simulink subsystem "VehicleElectroThermal"  (R2023a)
settings: Solver=VariableStepAuto  StartTime=0.0  StopTime=10.0  RelTol=1e-3
undefined symbols (not defined in the file): battery, cabin_T_init, coolant_pipe_D, coolant_valve_D_ratio_max, coolant_valve_D_ratio_min, coolant_valve_displacement, vehicleThermal
libraries: fl_lib x199, nesl_utility x54, SimscapeFluids_lib x15, ee_lib x9, sdl_lib x8, slpidlib x3, simulink x2, EmotorLib x2, BatteryCurrentManagement x1
(part 2 of 6)

== system VehicleElectroThermal/DCDC ==
  Coolant Jacket : SimscapeFluids_lib/Thermal Liquid/Pipes & Fittings/Pipe (TL)  dynamic_compressibility=1  inertia=0  num_segments=1  pipe_length=0.2 m  cross_section_geometry=fluids.thermal_liquid.pipes_fittings.enum.CrossSectionGeometry.Custom  pipe_diameter=0.1 m  pipe_inner_diameter=0.05 m  pipe_outer_diameter=0.1 m  pipe_width=0.1 m  pipe_height=0.1 m  pipe_major_axis=0.1 m  pipe_minor_axis=0.05 m  pipe_side=0.1 m  pipe_angle=30 deg  area=pi * vehicleThermal.coolant_channel_D^2 / 4 m^2  Dh=vehicleThermal.coolant_channel_D m  wall_spec=1  wall_compliance=1.2e-6 m/MPa  wall_time_constant=0.01 s  elevation_spec=foundation.enum.constant_variable.constant  elevation_gain=0 m  g=9.81 m/s^2  pressure_loss_spec=1  local_pressure_loss_spec=fluids.thermal_liquid.pipes_fittings.enum.LocalLossSpec.AggregateLength  length_add=0 m  loss_coefficient=0.1  roughness_spec=fluids.thermal_liquid.pipes_fittings.enum.RoughnessSpec.Custom  roughness=1.5e-5 m  Re_friction_TLU=[ 400 1000 1.5e+3 3e+3 4e+3 6e+3 1e+4 2e+4 4e+4 6e+4 1e+5 1e+8 ]  friction_factor_TLU=[ 0.264 0.112 0.07099999999999999 0.0417 0.0387 0.0268 0.025 0.0232 0.0226 0.022 0.0214 0.0214 ]  shape_factor=64  Re_lam=100  Re_tur=500  mdot_nominal=[ 0.1 1 ] kg/s  p_diff_nominal=[ 0.001 0.01 ] MPa  mdot_threshold=1e-6 kg/s  heat_transfer_spec=4  mdot_nominal_heat=[ 0.1 1 ] kg/s  T_in_nominal=[ 293.15 293.15 ] K  T_out_nominal=[ 300 300 ] K  p_in_nominal_heat=[ 0.101325 0.101325 ] MPa  T_wall_nominal=[ 303.15 303.15 ] K  a_coeff=0.3  b_Re_power=0.8  c_Pr_power=0.33  Nu_lam=3.66  Re_Colburn_TLU=[ 100 150 1000 ]  Colburn_factor_TLU=[ 0.019 0.013 0.002 ]  Re_Nu_TLU=[ 100 150 1000 ]  Pr_Nu_TLU=[ 1 10 ]  Nu_TLU=[ 3.72 4.21; 3.75 4.44; 4.21 7.15 ]  p0_vec=vehicleThermal.coolant_p_init MPa  T0_vec=vehicleThermal.coolant_T_init K  mdot0=0.1 kg/s
  DC-DC Converter mass : fl_lib/Thermal/Thermal Elements/Thermal Mass  mass_type=foundation.enum.constant_variable.constant  mass=1 kg  sp_heat=447 J/kg/K  mass_min=1e-6 kg  num_ports=foundation.enum.numPorts2.one  m_specify=off  m_priority=High  m=1 kg  m_nominal_specify=off  m_nominal_unit=kg  m_nominal_value=1  T_specify=on  T_priority=High  T=vehicleThermal.coolant_T_init K  T_nominal_specify=off  T_nominal_unit=K  T_nominal_value=1  Q_specify=off  Q_priority=None  Q=0 W  Q_nominal_specify=off  Q_nominal_unit=W  Q_nominal_value=1
  DC-DC Converter : ee_lib/Semiconductors & Converters/Converters/DC-DC Converter  Vref_option=ee.enum.converters.voltageref.internal  v_ref=100 V  P_rated=10000 W  droop_enabled=false  droop_param=ee.enum.converters.droop.value  droop=0.1 V/A  droop_percent=2  Vref_droop=10 V  reversible=ee.enum.converters.directionality.unidirectional  G_diode=1e-8 1/Ohm  P_fixed=1 W  losses_option=ee.enum.converters.lossesOption.proportionalToSquaredCurrent  eff_rated=80  tableOption=ee.enum.converters.lossTableOptionThermal.currentTemp  i_eff_vec=[-2, -1, 1, 2] A  v_eff_vec=[15, 30, 45] V  eff_vec=[66, 76, 80, 74]  eff_2D_table=[66, 66, 66; 76, 76, 76; 80, 80, 80; 74, 74, 74]  model_dynamics=ee.enum.converters.dynamics.yes  tau=0.02 s  v_ini=10 V  v1_min=1 V  R1=1000 Ohm  R2=1000 Ohm  enable_fault=simscape.enum.onoff.off  fault_condition=ee.enum.faults.faultInputCondition.greaterThan  fault_threshold=0.5  T_eff_vec=[280, 300, 320] K  eff_3D_table=repmat([66; 76; 80; 74], 1, 3, 3)  thermal_mass=100 J/K  initial_temperature=298.15 K
      settings: InternalSimscapePortConfiguration="{\"Bottom\":[],\"Left\":[{\"id\":\"p1\",\"label\":\"1+\",\"type\":\"foundation.electrical.electrical\"},{\"id\":\"n1\",\"label\":\"1-\",\"type\":\"foundation.electrical.electrical\"}],\"Right\":[{\"id\":\"p2\",\"label\":\"2+\",\"type\":\"foundation.electrical.electrical\"},{\"id\":\"n2\",\"label\":\"2-\",\"type\":\"foundation.electrical.electrical\"}],\"Top\":[]}"
  Electrical Reference : fl_lib/Electrical/Electrical Elements/Electrical Reference
  Electrical Reference1 : fl_lib/Electrical/Electrical Elements/Electrical Reference
  Flow Resistance (TL) : fl_lib/Thermal Liquid/Elements/Flow Resistance (TL)  delta_p_nominal=2e-3 MPa  mdot_nominal=0.02 kg/s  area=pi * vehicleThermal.coolant_pipe_D^2 / 4 m^2  laminar_fraction=1e-3
  Flow Resistance (TL)1 : fl_lib/Thermal Liquid/Elements/Flow Resistance (TL)  delta_p_nominal=1e-5 MPa  mdot_nominal=0.02 kg/s  area=pi * vehicleThermal.coolant_pipe_D^2 / 4 m^2  laminar_fraction=1e-3
  Heat Flow Source : fl_lib/Thermal/Thermal Sources/Controlled Heat Flow Rate Source
  PS Constant : fl_lib/Physical Signals/Sources/PS Constant  constant=0
  Thermal Reference : fl_lib/Thermal/Thermal Elements/Thermal Reference
  LV : PMIOPort  Side=Right
  B : PMIOPort  Port=2  Side=Right
  HV : PMIOPort  Port=3  Side=Right
  A : PMIOPort  Port=4  Side=Right
  connections:
  HV/RConn1 -- DC-DC Converter/LConn1
  DC-DC Converter/RConn1 -- LV/RConn1
  Coolant Jacket/LConn2 -- Heat Flow Source/LConn1 -- DC-DC Converter mass/LConn1
  Flow Resistance (TL)1/LConn1 -- A/RConn1
  DC-DC Converter/LConn2 -- Electrical Reference1/LConn1
  Flow Resistance (TL)1/RConn1 -- Coolant Jacket/RConn1
  Electrical Reference/LConn1 -- DC-DC Converter/RConn2
  Flow Resistance (TL)/LConn1 -- Coolant Jacket/LConn1
  Flow Resistance (TL)/RConn1 -- B/RConn1
  Thermal Reference/LConn1 -- Heat Flow Source/RConn2
  PS Constant/RConn1 -- Heat Flow Source/RConn1

== system VehicleElectroThermal/Driveline ==
  s : Inport
  Brake Rear : sdl_lib/Brakes & Detents/Rotational/Disc Brake  r_mean=150 mm  bore=10 mm  n_pads=2  thermal_port=simscape.enum.thermaleffects.omit  mu_static=0.9  mu_coulomb=0.7  temperature_TLU=[280, 300, 320] K  mu_static_TLU=[.9, .8, .7]  mu_coulomb_TLU=[.8, .7, .6]  brkwy_vel=0.1 rad/s  visc_coef=0 N*m*s/rad  enable_faults=simscape.enum.onoff.off  faulted_pressure=0 bar  external_fault=simscape.enum.onoff.off  temporal_fault=simscape.enum.onoff.off  fault_time=5 s  report_fault=simscape.enum.assert.action.none  thermal_mass=50 kJ/K  temperature_specify=off  temperature_priority=High  temperature=300 K  temperature_nominal_specify=off  temperature_nominal_unit=K  temperature_nominal_value=1
  PS-Simulink Converter1 : nesl_utility/PS-Simulink Converter  PhysicalDomain=network_engine_domain  SubClassName=ps_output  LeftPortType=input  RightPortType=output  PseudoPeriodic=off  Frequencies=[]  VectorFormat=inherit  Unit=km/hr  AffineConversion=off
  Simulink-PS Converter1 : nesl_utility/Simulink-PS Converter  PhysicalDomain=network_engine_domain  SubClassName=ps_input  LeftPortType=input  RightPortType=output  PseudoPeriodic=off  Frequencies=[]  NoiseDistribution=none  NoiseParameters=[]  Unit=1  AffineConversion=off  FilteringAndDerivatives=provide  SimscapeFilterOrder=1  InputFilterTimeConstant=0.001  UdotUserProvided=0
  Tire FL : sdl_lib/Tires & Vehicles/Tire (Magic Formula)  parameterization=sdl.enum.magic_tire_model.peak  F_z1=3000 N  F_x1=3500 N  kappa1=10  B_m=10  C_m=1.9  D_m=1  E_m=0.97  fz0=4000 N  p_Cx=1.685  p_Dx=[1.21, -.037]  p_Ex=[.344, .095, -.02, 0]  p_Kx=[21.51, -.163, .245]  p_Hx=[-.002, .002]  p_Vx=[0, 0]  rolling_radius_model=sdl.enum.RollingRadiusParameterization.Constant  r_e="vehicle.tireRollingRadius_cm  cm"  r_0=0.3 m  breff=8.39  dreff=0.26  freff=0.074  q_re0=0.99  q_v1=0.008  longvl=17 m/s  cz=5e5 N/m  model_resistance=simscape.enum.onoff.off  resistance_model=sdl.enum.rollingResistanceParameterization.constant  coeff=0.015  p_tire=250e3 Pa  alpha=-0.003  beta=0.97  coeff_a=84e-4  coeff_b=6.2e-4 s/m  coeff_c=1.6e-4 s^2/m^2  p_tire0=240e3 Pa  fz0_resistance=4000 N  vH0=16 m/s  q_Sy=[.0082, 0, .0014, .001, 0, 0, 1.08, -.5]  v_thr=0.001 m/s  enable_scaling_coefficients=false  lfzO=1  lcx=1  lmux=1  lex=1  lkx=1  lhx=1  lvx=1  lmy=1  model_compliance=sdl.enum.compliance.off  stiffness=1e6 N/m  damping=1000 N*s/m  model_inertia=sdl.enum.model_inertia.off  inertia=1 kg*m^2  initial_velocity=0 rad/s  vxlow=0.1 m/s  v_tr_thr=0.1*(0.1) m/s  kpumin=-1e5  kpumax=1e5
  Tire FR : sdl_lib/Tires & Vehicles/Tire (Magic Formula)  parameterization=sdl.enum.magic_tire_model.peak  F_z1=3000 N  F_x1=3500 N  kappa1=10  B_m=10  C_m=1.9  D_m=1  E_m=0.97  fz0=4000 N  p_Cx=1.685  p_Dx=[1.21, -.037]  p_Ex=[.344, .095, -.02, 0]  p_Kx=[21.51, -.163, .245]  p_Hx=[-.002, .002]  p_Vx=[0, 0]  rolling_radius_model=sdl.enum.RollingRadiusParameterization.Constant  r_e="vehicle.tireRollingRadius_cm  cm"  r_0=0.3 m  breff=8.39  dreff=0.26  freff=0.074  q_re0=0.99  q_v1=0.008  longvl=17 m/s  cz=5e5 N/m  model_resistance=simscape.enum.onoff.off  resistance_model=sdl.enum.rollingResistanceParameterization.constant  coeff=0.015  p_tire=250e3 Pa  alpha=-0.003  beta=0.97  coeff_a=84e-4  coeff_b=6.2e-4 s/m  coeff_c=1.6e-4 s^2/m^2  p_tire0=240e3 Pa  fz0_resistance=4000 N  vH0=16 m/s  q_Sy=[.0082, 0, .0014, .001, 0, 0, 1.08, -.5]  v_thr=0.001 m/s  enable_scaling_coefficients=false  lfzO=1  lcx=1  lmux=1  lex=1  lkx=1  lhx=1  lvx=1  lmy=1  model_compliance=sdl.enum.compliance.off  stiffness=1e6 N/m  damping=1000 N*s/m  model_inertia=sdl.enum.model_inertia.off  inertia=1 kg*m^2  initial_velocity=0 rad/s  vxlow=0.1 m/s  v_tr_thr=0.1*(0.1) m/s  kpumin=-1e5  kpumax=1e5
  Tire RL : sdl_lib/Tires & Vehicles/Tire (Magic Formula)  parameterization=sdl.enum.magic_tire_model.peak  F_z1=3000 N  F_x1=3500 N  kappa1=10  B_m=10  C_m=1.9  D_m=1  E_m=0.97  fz0=4000 N  p_Cx=1.685  p_Dx=[1.21, -.037]  p_Ex=[.344, .095, -.02, 0]  p_Kx=[21.51, -.163, .245]  p_Hx=[-.002, .002]  p_Vx=[0, 0]  rolling_radius_model=sdl.enum.RollingRadiusParameterization.Constant  r_e="vehicle.tireRollingRadius_cm  cm"  r_0=0.3 m  breff=8.39  dreff=0.26  freff=0.074  q_re0=0.99  q_v1=0.008  longvl=17 m/s  cz=5e5 N/m  model_resistance=simscape.enum.onoff.off  resistance_model=sdl.enum.rollingResistanceParameterization.constant  coeff=0.015  p_tire=250e3 Pa  alpha=-0.003  beta=0.97  coeff_a=84e-4  coeff_b=6.2e-4 s/m  coeff_c=1.6e-4 s^2/m^2  p_tire0=240e3 Pa  fz0_resistance=4000 N  vH0=16 m/s  q_Sy=[.0082, 0, .0014, .001, 0, 0, 1.08, -.5]  v_thr=0.001 m/s  enable_scaling_coefficients=false  lfzO=1  lcx=1  lmux=1  lex=1  lkx=1  lhx=1  lvx=1  lmy=1  model_compliance=sdl.enum.compliance.off  stiffness=1e6 N/m  damping=1000 N*s/m  model_inertia=sdl.enum.model_inertia.off  inertia=1 kg*m^2  initial_velocity=0 rad/s  vxlow=0.1 m/s  v_tr_thr=0.1*(0.1) m/s  kpumin=-1e5  kpumax=1e5
  Tire RR : sdl_lib/Tires & Vehicles/Tire (Magic Formula)  parameterization=sdl.enum.magic_tire_model.peak  F_z1=3000 N  F_x1=3500 N  kappa1=10  B_m=10  C_m=1.9  D_m=1  E_m=0.97  fz0=4000 N  p_Cx=1.685  p_Dx=[1.21, -.037]  p_Ex=[.344, .095, -.02, 0]  p_Kx=[21.51, -.163, .245]  p_Hx=[-.002, .002]  p_Vx=[0, 0]  rolling_radius_model=sdl.enum.RollingRadiusParameterization.Constant  r_e="vehicle.tireRollingRadius_cm  cm"  r_0=0.3 m  breff=8.39  dreff=0.26  freff=0.074  q_re0=0.99  q_v1=0.008  longvl=17 m/s  cz=5e5 N/m  model_resistance=simscape.enum.onoff.off  resistance_model=sdl.enum.rollingResistanceParameterization.constant  coeff=0.015  p_tire=250e3 Pa  alpha=-0.003  beta=0.97  coeff_a=84e-4  coeff_b=6.2e-4 s/m  coeff_c=1.6e-4 s^2/m^2  p_tire0=240e3 Pa  fz0_resistance=4000 N  vH0=16 m/s  q_Sy=[.0082, 0, .0014, .001, 0, 0, 1.08, -.5]  v_thr=0.001 m/s  enable_scaling_coefficients=false  lfzO=1  lcx=1  lmux=1  lex=1  lkx=1  lhx=1  lvx=1  lmy=1  model_compliance=sdl.enum.compliance.off  stiffness=1e6 N/m  damping=1000 N*s/m  model_inertia=sdl.enum.model_inertia.off  inertia=1 kg*m^2  initial_velocity=0 rad/s  vxlow=0.1 m/s  v_tr_thr=0.1*(0.1) m/s  kpumin=-1e5  kpumax=1e5
  Vehicle Body : sdl_lib/Tires & Vehicles/Vehicle Body  mass=vehicle.vehMass_kg kg  n_w=2  x_f=1.4 m  x_r=1.6 m  y_c=0.5 m  mass_var=simscape.enum.onoff.off  g=9.81 m/s^2  liftoff_warning=simscape.enum.onoff.off  area=3 m^2  Cd=0.4  rho=1.18 kg/m^3  model_pitch=simscape.enum.onoff.off  inertia=4000 kg*m^2  suspension_model=sdl.enum.linearTLU.linear  k_f=1e4 N/m  b_f=1e4 N*s/m  k_r=1e4 N/m  b_r=1e4 N*s/m  k_f_TLU=[-2000, -1000, 0, 1000, 2000] N  x_f_TLU=[-.4, -.2, 0, .2, .4] m  b_f_TLU=[-200, -100, 0, 100, 200] N  v_f_TLU=[-4, -2, 0, 2, 4] m/s  k_r_TLU=[-2000, -1000, 0, 1000, 2000] N  x_r_TLU=[-.4, -.2, 0, .2, .4] m  b_r_TLU=[-200, -100, 0, 100, 200] N  v_r_TLU=[-4, -2, 0, 2, 4] m/s  interp_method=simscape.enum.interpolation.linear  extrap_method=simscape.enum.extrapolation.linear  model_hardstop=simscape.enum.onoff.off  upper_bound_f=.25 m  lower_bound_f=-.25 m  stop_k_f=1e6 N/m  stop_b_f=150 N*s/m  upper_bound_r=.25 m  lower_bound_r=-.25 m  stop_k_r=1e6 N/m  stop_b_r=150 N*s/m  initial_pitch=0 rad  initial_pitch_rate=0 rad/s  v_specify=on  v_priority=High  v=0 kph  v_nominal_specify=on  v_nominal_unit=m/s  v_nominal_value=1
  FA : PMIOPort  Side=Left
  RA : PMIOPort  Port=2  Side=Right
  Bus Element Out : Outport  PortName=m  Element=VehSpd
  wires:
  s/1 -> [BrkCmd]
  PS-Simulink Converter1/1 -> Bus Element Out/1  "VehSpd"
  [BrkCmd] -> Simulink-PS Converter1/1
  connections:
  Tire FL/LConn1 -- Tire FR/LConn1 -- Vehicle Body/RConn2
  Tire RR/LConn1 -- Vehicle Body/RConn1 -- Tire RL/LConn1
  PS-Simulink Converter1/LConn1 -- Vehicle Body/LConn2
  Tire FR/LConn2 -- FA/RConn1 -- Tire FL/LConn2
  Brake Rear/LConn2 -- RA/RConn1 -- Tire RR/LConn2 -- Tire RL/LConn2
  Tire FL/RConn2 -- Vehicle Body/LConn1 -- Tire RR/RConn2 -- Tire RL/RConn2 -- Tire FR/RConn2
  Simulink-PS Converter1/RConn1 -- Brake Rear/LConn1

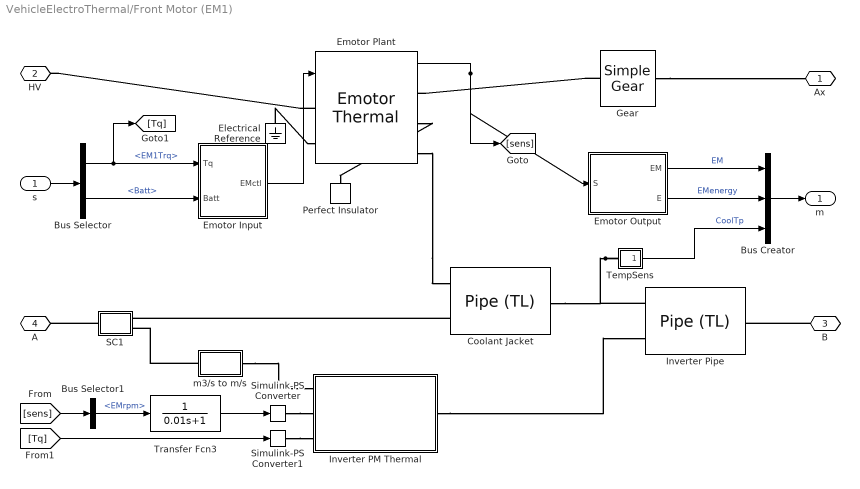
== system VehicleElectroThermal/Front Motor (EM1) ==
  s : Inport
  Bus Creator : BusCreator  Inputs=3
  Bus Selector : BusSelector  OutputSignals=EM1Trq,Batt
  Bus Selector1 : BusSelector  OutputSignals=EMrpm
  Coolant Jacket : SimscapeFluids_lib/Thermal Liquid/Pipes & Fittings/Pipe (TL)  dynamic_compressibility=1  inertia=0  num_segments=1  pipe_length=0.4 m  cross_section_geometry=fluids.thermal_liquid.pipes_fittings.enum.CrossSectionGeometry.Custom  pipe_diameter=0.1 m  pipe_inner_diameter=0.05 m  pipe_outer_diameter=0.1 m  pipe_width=0.1 m  pipe_height=0.1 m  pipe_major_axis=0.1 m  pipe_minor_axis=0.05 m  pipe_side=0.1 m  pipe_angle=30 deg  area=4 * pi * vehicleThermal.coolant_channel_D^2 / 4 m^2  Dh=vehicleThermal.coolant_channel_D m  wall_spec=1  wall_compliance=1.2e-6 m/MPa  wall_time_constant=0.01 s  elevation_spec=foundation.enum.constant_variable.constant  elevation_gain=0 m  g=9.81 m/s^2  pressure_loss_spec=1  local_pressure_loss_spec=fluids.thermal_liquid.pipes_fittings.enum.LocalLossSpec.AggregateLength  length_add=20 * vehicleThermal.coolant_channel_D * 4 m  loss_coefficient=0.1  roughness_spec=fluids.thermal_liquid.pipes_fittings.enum.RoughnessSpec.Custom  roughness=1.5e-5 m  Re_friction_TLU=[ 400 1000 1.5e+3 3e+3 4e+3 6e+3 1e+4 2e+4 4e+4 6e+4 1e+5 1e+8 ]  friction_factor_TLU=[ 0.264 0.112 0.07099999999999999 0.0417 0.0387 0.0268 0.025 0.0232 0.0226 0.022 0.0214 0.0214 ]  shape_factor=64  Re_lam=100  Re_tur=500  mdot_nominal=[ 0.1 1 ] kg/s  p_diff_nominal=[ 0.001 0.01 ] MPa  mdot_threshold=1e-6 kg/s  heat_transfer_spec=4  mdot_nominal_heat=[ 0.1 1 ] kg/s  T_in_nominal=[ 293.15 293.15 ] K  T_out_nominal=[ 300 300 ] K  p_in_nominal_heat=[ 0.101325 0.101325 ] MPa  T_wall_nominal=[ 303.15 303.15 ] K  a_coeff=0.3  b_Re_power=0.8  c_Pr_power=0.33  Nu_lam=3.66  Re_Colburn_TLU=[ 100 150 1000 ]  Colburn_factor_TLU=[ 0.019 0.013 0.002 ]  Re_Nu_TLU=[ 100 150 1000 ]  Pr_Nu_TLU=[ 1 10 ]  Nu_TLU=[ 3.72 4.21; 3.75 4.44; 4.21 7.15 ]  p0_vec=vehicleThermal.coolant_p_init MPa  T0_vec=vehicleThermal.coolant_T_init K  mdot0=0.1 kg/s
  Electrical Reference : fl_lib/Electrical/Electrical Elements/Electrical Reference
  Emotor Input : Subsystem
  Emotor Output : Subsystem
  Emotor Plant : EmotorLib/Emotor Thermal  InitTemp=vehicleThermal.coolant_T_init  IronSpHeat=electricDrive.IronSpHeat  CopperSpHeat=electricDrive.CopperSpHeat  IronThConductivity=electricDrive.IronThConductivity  GrossToothMass=electricDrive.MotorThermal.GrossToothMass  WindingMass=electricDrive.MotorThermal.WindingMass  max_torque=electricDrive.max_torque  max_power=electricDrive.max_power  Tctc=electricDrive.Tctc  spMat=electricDrive.motor_loss_map.spMat  tqMat=electricDrive.motor_loss_map.tqMat  lossMat=electricDrive.motor_loss_map.lossMat  StatorBackIronMass=electricDrive.MotorThermal.StatorBackIronMass  StatorRootDia=electricDrive.MotorThermal.StatorRootDia  stator_od=electricDrive.MotorThermal.stator_od  StatorWindingOhArea=electricDrive.MotorThermal.StatorWindingOhArea  Bridgemass=electricDrive.MotorThermal.Bridgemass  rotor_od=electricDrive.MotorThermal.rotor_od  rotorStackLength=electricDrive.MotorThermal.rotorStackLength  RotorBackIronMass=electricDrive.MotorThermal.RotorBackIronMass  RotorAreaER=electricDrive.MotorThermal.RotorAreaER  RotorAreaCyl=electricDrive.MotorThermal.RotorAreaCyl
  Gear : sdl_lib/Gears/Simple Gear  ratio=10/3  rotation_direction=sdl.enum.shaftOutputDirection.same  friction_model=sdl.enum.gear_efficiencies_load.off  T_noload=0.1 N*m  T_nom=5 N*m  efficiency_nom=0.8  efficiency=0.8  temperature_TLU=[280, 300, 320] K  load_TLU=[1, 5, 10] N*m  efficiency_TLU=[.95, .9, .85]  efficiency_TLU2=[.85, .8, .75; .95, .9, .85; .85, .8, .7]  w_thr=0.01 rad/s  pwr_thr=0.001 W  enable_backlash=false  hardstop_model=simscape.enum.hardstop.smooth  backlash_distance=1e-3 mm  r_base=0.1 m  transition=1e-4 mm  backlash_stiffness=1e7 N/m  backlash_damping=1e6 N*s/m  coeff_rest=0  v_tol=0.001 m/s  f_tol=0 N  mu_visc=[0, 0] N*m*s/rad  enable_faults=simscape.enum.onoff.off  efficiency_fault=0.05  external_fault=simscape.enum.onoff.off  temporal_fault=simscape.enum.onoff.off  fault_time=5 s  fault_angles=pi / 12 rad  report_fault=simscape.enum.assert.action.none  thermal_mass=50 J/K  temperature_specify=off  temperature_priority=High  temperature=300 K  temperature_nominal_specify=off  temperature_nominal_unit=K  temperature_nominal_value=1  x_backlash_specify=off  x_backlash_priority=None  x_backlash=0 mm  x_backlash_nominal_specify=off  x_backlash_nominal_unit=mm  x_backlash_nominal_value=1  f_hardstop_specify=off  f_hardstop_priority=None  f_hardstop=0 N  f_hardstop_nominal_specify=off  f_hardstop_nominal_unit=N  f_hardstop_nominal_value=1  v_backlash_specify=off  v_backlash_priority=None  v_backlash=0 m/s  v_backlash_nominal_specify=off  v_backlash_nominal_unit=m/s  v_backlash_nominal_value=1
  Inverter PM Thermal : Subsystem
  Inverter Pipe : SimscapeFluids_lib/Thermal Liquid/Pipes & Fittings/Pipe (TL)  dynamic_compressibility=1  inertia=0  num_segments=1  pipe_length=0.4 m  cross_section_geometry=fluids.thermal_liquid.pipes_fittings.enum.CrossSectionGeometry.Custom  pipe_diameter=0.1 m  pipe_inner_diameter=0.05 m  pipe_outer_diameter=0.1 m  pipe_width=0.1 m  pipe_height=0.1 m  pipe_major_axis=0.1 m  pipe_minor_axis=0.05 m  pipe_side=0.1 m  pipe_angle=30 deg  area=4 * pi * vehicleThermal.coolant_channel_D^2 / 4 m^2  Dh=vehicleThermal.coolant_channel_D m  wall_spec=1  wall_compliance=1.2e-6 m/MPa  wall_time_constant=0.01 s  elevation_spec=foundation.enum.constant_variable.constant  elevation_gain=0 m  g=9.81 m/s^2  pressure_loss_spec=1  local_pressure_loss_spec=fluids.thermal_liquid.pipes_fittings.enum.LocalLossSpec.AggregateLength  length_add=20 * vehicleThermal.coolant_channel_D * 4 m  loss_coefficient=0.1  roughness_spec=fluids.thermal_liquid.pipes_fittings.enum.RoughnessSpec.Custom  roughness=1.5e-5 m  Re_friction_TLU=[ 400 1000 1.5e+3 3e+3 4e+3 6e+3 1e+4 2e+4 4e+4 6e+4 1e+5 1e+8 ]  friction_factor_TLU=[ 0.264 0.112 0.07099999999999999 0.0417 0.0387 0.0268 0.025 0.0232 0.0226 0.022 0.0214 0.0214 ]  shape_factor=64  Re_lam=100  Re_tur=500  mdot_nominal=[ 0.1 1 ] kg/s  p_diff_nominal=[ 0.001 0.01 ] MPa  mdot_threshold=1e-6 kg/s  heat_transfer_spec=4  mdot_nominal_heat=[ 0.1 1 ] kg/s  T_in_nominal=[ 293.15 293.15 ] K  T_out_nominal=[ 300 300 ] K  p_in_nominal_heat=[ 0.101325 0.101325 ] MPa  T_wall_nominal=[ 303.15 303.15 ] K  a_coeff=0.3  b_Re_power=0.8  c_Pr_power=0.33  Nu_lam=3.66  Re_Colburn_TLU=[ 100 150 1000 ]  Colburn_factor_TLU=[ 0.019 0.013 0.002 ]  Re_Nu_TLU=[ 100 150 1000 ]  Pr_Nu_TLU=[ 1 10 ]  Nu_TLU=[ 3.72 4.21; 3.75 4.44; 4.21 7.15 ]  p0_vec=vehicleThermal.coolant_p_init MPa  T0_vec=vehicleThermal.coolant_T_init K  mdot0=0.1 kg/s
  Perfect Insulator : fl_lib/Thermal/Thermal Elements/Perfect Insulator  T_specify=off  T_priority=None  T=293.15 K  T_nominal_specify=off  T_nominal_unit=K  T_nominal_value=1
  SC1 : Subsystem
      mask Display: disp(get_param(gcb, 'Name'))
  Simulink-PS Converter : nesl_utility/Simulink-PS Converter  PhysicalDomain=network_engine_domain  SubClassName=ps_input  LeftPortType=input  RightPortType=output  PseudoPeriodic=off  Frequencies=[]  NoiseDistribution=none  NoiseParameters=[]  Unit=rpm  AffineConversion=off  FilteringAndDerivatives=provide  SimscapeFilterOrder=1  InputFilterTimeConstant=0.001  UdotUserProvided=0
  Simulink-PS Converter1 : nesl_utility/Simulink-PS Converter  PhysicalDomain=network_engine_domain  SubClassName=ps_input  LeftPortType=input  RightPortType=output  PseudoPeriodic=off  Frequencies=[]  NoiseDistribution=none  NoiseParameters=[]  Unit=N*m  AffineConversion=off  FilteringAndDerivatives=provide  SimscapeFilterOrder=1  InputFilterTimeConstant=0.001  UdotUserProvided=0
  TempSens : Subsystem
  Transfer Fcn3 : TransferFcn  Denominator=[0.01 1]
  m3/s to m/s : Subsystem
  Ax : PMIOPort  Side=Left
  HV : PMIOPort  Port=2  Side=Right
  B : PMIOPort  Port=3  Side=Right
  A : PMIOPort  Port=4  Side=Right
  m : Outport
  wires:
  s/1 -> Bus Selector/1
  Transfer Fcn3/1 -> Simulink-PS Converter/1
  [Tq] -> Simulink-PS Converter1/1
  Bus Selector1/1 -> Transfer Fcn3/1  "<EMrpm>"
  [sens] -> Bus Selector1/1
  Bus Creator/1 -> m/1
  TempSens/1("  ") -> Bus Creator/3  "CoolTp"
  Emotor Output/2(E) -> Bus Creator/2  "EMenergy"
  Emotor Output/1(EM) -> Bus Creator/1  "EM"
  Emotor Plant/1 -> [sens], Emotor Output/1(S)
  Emotor Input/1(EMctl) -> Emotor Plant/1
  Bus Selector/2 -> Emotor Input/2("Batt ")  "<Batt>"
  Bus Selector/1 -> Emotor Input/1("Tq  "), [Tq]  "<EM1Trq>"
  connections:
  Electrical Reference/LConn1 -- Emotor Plant/LConn2
  Gear/LConn1 -- Emotor Plant/RConn1
  Emotor Plant/RConn2 -- Perfect Insulator/LConn1
  m3/s to m/s/LConn1 -- SC1/RConn2
  m3/s to m/s/RConn1 -- Inverter PM Thermal/LConn1
  SC1/LConn1 -- A/RConn1
  Simulink-PS Converter1/RConn1 -- Inverter PM Thermal/LConn3
  Simulink-PS Converter/RConn1 -- Inverter PM Thermal/LConn2
  Inverter PM Thermal/RConn1 -- Inverter Pipe/LConn2
  B/RConn1 -- Inverter Pipe/RConn1
  Emotor Plant/LConn1 -- HV/RConn1
  TempSens/LConn1 -- Inverter Pipe/LConn1 -- Coolant Jacket/RConn1
  Emotor Plant/RConn3 -- Coolant Jacket/LConn2
  Gear/RConn1 -- Ax/RConn1
  Coolant Jacket/LConn1 -- SC1/RConn1

== system VehicleElectroThermal/HVAC ==
  s : Inport
  Bus Selector : BusSelector  OutputSignals=Batt.BattSensor.BatVolt,Batt.BatSt,Tenv,TpSetPoint,acOnOff,Batt
  Cabin : Subsystem
  Controlled Current Source : fl_lib/Electrical/Electrical Sources/Controlled Current Source
  Electrical Reference : fl_lib/Electrical/Electrical Elements/Electrical Reference
  Electrical Reference1 : fl_lib/Electrical/Electrical Elements/Electrical Reference
  HVAC Demand : Subsystem
  HVAC Energy : Subsystem
  PS-Simulink Converter : nesl_utility/PS-Simulink Converter  PhysicalDomain=network_engine_domain  SubClassName=ps_output  LeftPortType=input  RightPortType=output  PseudoPeriodic=off  Frequencies=[]  VectorFormat=inherit  Unit=inherit  AffineConversion=off
  Simulink-PS Converter : nesl_utility/Simulink-PS Converter  PhysicalDomain=network_engine_domain  SubClassName=ps_input  LeftPortType=input  RightPortType=output  PseudoPeriodic=off  Frequencies=[]  NoiseDistribution=none  NoiseParameters=[]  Unit=1  AffineConversion=off  FilteringAndDerivatives=provide  SimscapeFilterOrder=1  InputFilterTimeConstant=0.001  UdotUserProvided=0
  Simulink-PS Converter1 : nesl_utility/Simulink-PS Converter  PhysicalDomain=network_engine_domain  SubClassName=ps_input  LeftPortType=input  RightPortType=output  PseudoPeriodic=off  Frequencies=[]  NoiseDistribution=none  NoiseParameters=[]  Unit=W  AffineConversion=off  FilteringAndDerivatives=provide  SimscapeFilterOrder=1  InputFilterTimeConstant=0.001  UdotUserProvided=0
  Simulink-PS Converter2 : nesl_utility/Simulink-PS Converter  PhysicalDomain=network_engine_domain  SubClassName=ps_input  LeftPortType=input  RightPortType=output  PseudoPeriodic=off  Frequencies=[]  NoiseDistribution=none  NoiseParameters=[]  Unit=W  AffineConversion=off  FilteringAndDerivatives=provide  SimscapeFilterOrder=1  InputFilterTimeConstant=0.001  UdotUserProvided=0
  Voltage Sensor : fl_lib/Electrical/Electrical Sensors/Voltage Sensor
  HV : PMIOPort  Side=Left
  Bus Element Out : Outport  PortName=m  Element=HVACenergy
  wires:
  Bus Selector/2 -> Simulink-PS Converter/1  "<BatSt>"
  Cabin/2(PTC) -> Simulink-PS Converter1/1
  Cabin/1(Cool) -> Simulink-PS Converter2/1
  Bus Selector/6 -> HVAC Energy/2(Batt)  "<Batt>"
  PS-Simulink Converter/1 -> HVAC Energy/1(I)
  Bus Selector/5 -> Cabin/3(acOnOff)  "<acOnOff>"
  Bus Selector/4 -> Cabin/2(Tsetpoint)  "<TpSetPoint>"
  Bus Selector/3 -> Cabin/1(Tenv)  "<Tenv>"
  s/1 -> Bus Selector/1
  HVAC Energy/1(E) -> Bus Element Out/1  "HVACenergy"
  connections:
  Electrical Reference1/LConn1 -- Voltage Sensor/RConn2
  Controlled Current Source/RConn1 -- PS-Simulink Converter/LConn1 -- HVAC Demand/RConn1
  Simulink-PS Converter1/RConn1 -- HVAC Demand/LConn4
  HVAC Demand/LConn3 -- Simulink-PS Converter2/RConn1
  Simulink-PS Converter/RConn1 -- HVAC Demand/LConn2
  Voltage Sensor/RConn1 -- HVAC Demand/LConn1
  Voltage Sensor/LConn1 -- Controlled Current Source/RConn2 -- HV/RConn1
  Controlled Current Source/LConn1 -- Electrical Reference/LConn1

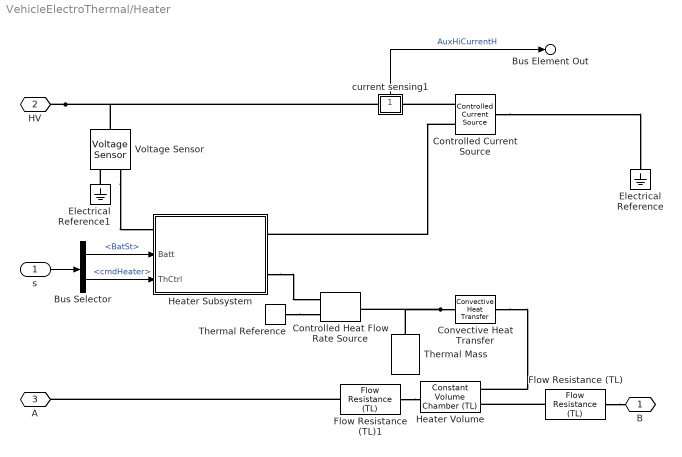
== system VehicleElectroThermal/Heater ==
  s : Inport
  Bus Selector : BusSelector  OutputSignals=BatSt,cmdHeater
  Controlled Current Source : fl_lib/Electrical/Electrical Sources/Controlled Current Source
  Controlled Heat Flow Rate Source : fl_lib/Thermal/Thermal Sources/Controlled Heat Flow Rate Source
  Convective Heat Transfer : fl_lib/Thermal/Thermal Elements/Convective Heat Transfer  thermal_type=foundation.enum.constant_variable.constant  area=1 m^2  heat_tr_coeff=200 W/(m^2 * K)  min_heat_tr_coeff=1e-3 W/(K*m^2)  T_specify=off  T_priority=None  T=0 K  T_nominal_specify=off  T_nominal_unit=K  T_nominal_value=1  Q_specify=off  Q_priority=None  Q=0 W  Q_nominal_specify=off  Q_nominal_unit=W  Q_nominal_value=1
  Electrical Reference : fl_lib/Electrical/Electrical Elements/Electrical Reference
  Electrical Reference1 : fl_lib/Electrical/Electrical Elements/Electrical Reference
  Flow Resistance (TL) : fl_lib/Thermal Liquid/Elements/Flow Resistance (TL)  delta_p_nominal=2e-4 MPa  mdot_nominal=0.15 kg/s  area=pi * vehicleThermal.coolant_pipe_D^2 / 4 m^2  laminar_fraction=1e-3
  Flow Resistance (TL)1 : fl_lib/Thermal Liquid/Elements/Flow Resistance (TL)  delta_p_nominal=2e-4 MPa  mdot_nominal=0.15 kg/s  area=pi * vehicleThermal.coolant_pipe_D^2 / 4 m^2  laminar_fraction=1e-3
  Heater Volume : fl_lib/Thermal Liquid/Elements/Constant Volume Chamber (TL)  volume=0.001 m^3  num_ports=foundation.enum.num_ports.two  area_A=pi * vehicleThermal.coolant_pipe_D^2 / 4 m^2  area_B=pi * vehicleThermal.coolant_pipe_D^2 / 4 m^2  area_C=0.01 m^2  area_D=0.01 m^2  p_I_specify=on  p_I_priority=High  p_I=vehicleThermal.coolant_p_init MPa  p_I_nominal_specify=off  p_I_nominal_unit=MPa  p_I_nominal_value=1  T_I_specify=on  T_I_priority=High  T_I=vehicleThermal.coolant_T_init K  T_I_nominal_specify=off  T_I_nominal_unit=K  T_I_nominal_value=1  u_I_specify=off  u_I_priority=None  u_I=83.90600000000001 kJ/kg  u_I_nominal_specify=off  u_I_nominal_unit=kJ/kg  u_I_nominal_value=1  rho_I_specify=off  rho_I_priority=None  rho_I=998.21 kg/m^3  rho_I_nominal_specify=off  rho_I_nominal_unit=kg/m^3  rho_I_nominal_value=1
      settings: InternalSimscapePortConfiguration="{\"Bottom\":[],\"Left\":[{\"id\":\"A\",\"label\":\"A\",\"type\":\"foundation.thermal_liquid.thermal_liquid\"},{\"id\":\"H\",\"label\":\"H\",\"type\":\"foundation.thermal.thermal\"}],\"Right\":[{\"id\":\"B\",\"label\":\"B\",\"type\":\"foundation.thermal_liquid.thermal_liquid\"}],\"Top\":[]}"
  Heater Subsystem : Subsystem
      settings: PortSchema="{\"entries\":[{\"content\":{\"sides\":[{\"content\":{\"connectorIds\":[\"LConn1\",\"In1\",\"In2\"]},\"type\":\"ConnectorPlacement.EquallySpacedRectSide\",\"uuid\":\"d995acd0-973b-4873-b050-eaa71c2c53f5\"},{\"content\":{\"connectorIds\":[\"RConn1\",\"RConn2\"],\"side\":\"RIGHT\"},\"type\":\"ConnectorPlacement.EquallySpacedRectSide\",\"uuid\":\"f40dc2d9-a9a2-427c-8e3f-65ba63c73559\"},{\"content\":{\"connectorIds\":[],\"side\":\"TOP\"},\"type\":\"ConnectorPlacement.EquallySpacedRectSide\",\"uuid\":\"1868aaf5-b9f5-4fdb-94e9-4b9189d403a5\"}]},\"type\":\"ConnectorPlacement.EquallySpacedConnector\",\"uuid\":\"c13a0ccf-549d-47cf-8e66-a96ce55255c8\"}],\"packageUris\":[\"http://schema.mathworks.com/mf0/Connector/R2020b\"],\"version\":\"1.0\"}"
  Thermal Mass : fl_lib/Thermal/Thermal Elements/Thermal Mass  mass_type=foundation.enum.constant_variable.constant  mass=2 kg  sp_heat=447 J/kg/K  mass_min=1e-6 kg  num_ports=foundation.enum.numPorts2.one  m_specify=off  m_priority=High  m=1 kg  m_nominal_specify=off  m_nominal_unit=kg  m_nominal_value=1  T_specify=on  T_priority=High  T=vehicleThermal.coolant_T_init K  T_nominal_specify=off  T_nominal_unit=K  T_nominal_value=1  Q_specify=off  Q_priority=None  Q=0 W  Q_nominal_specify=off  Q_nominal_unit=W  Q_nominal_value=1
  Thermal Reference : fl_lib/Thermal/Thermal Elements/Thermal Reference
  Voltage Sensor : fl_lib/Electrical/Electrical Sensors/Voltage Sensor
  current sensing1 : Subsystem
      settings: PortSchema="{\"entries\":[{\"content\":{\"sides\":[{\"content\":{\"connectorIds\":[\"LConn1\"]},\"type\":\"ConnectorPlacement.EquallySpacedRectSide\",\"uuid\":\"be2815b5-7c4b-4452-9f46-9765620d338b\"},{\"content\":{\"connectorIds\":[\"RConn1\"],\"side\":\"RIGHT\"},\"type\":\"ConnectorPlacement.EquallySpacedRectSide\",\"uuid\":\"398ebab2-f4fa-4d00-bf6e-74bf1f6972c5\"},{\"content\":{\"connectorIds\":[\"Out1\"],\"side\":\"TOP\"},\"type\":\"ConnectorPlacement.EquallySpacedRectSide\",\"uuid\":\"f18d5713-17ec-4be9-9072-3e03c5a4f599\"}]},\"type\":\"ConnectorPlacement.EquallySpacedConnector\",\"uuid\":\"966ec05e-6316-4039-8e26-1d6b096cf423\"}],\"packageUris\":[\"http://schema.mathworks.com/mf0/Connector/R2020b\"],\"version\":\"1.0\"}"
  B : PMIOPort  Side=Right
  HV : PMIOPort  Port=2  Side=Right
  A : PMIOPort  Port=3  Side=Right
  Bus Element Out : Outport  PortName=m  Element=HeaterCurrent
  wires:
  s/1 -> Bus Selector/1
  Bus Selector/2 -> Heater Subsystem/2(ThCtrl)  "<cmdHeater>"
  Bus Selector/1 -> Heater Subsystem/1(Batt)  "<BatSt>"
  current sensing1/1("   ") -> Bus Element Out/1  "AuxHiCurrentH"
  connections:
  Voltage Sensor/RConn1 -- Heater Subsystem/LConn1
  Electrical Reference1/LConn1 -- Voltage Sensor/RConn2
  Controlled Current Source/RConn1 -- Heater Subsystem/RConn1
  Convective Heat Transfer/LConn1 -- Controlled Heat Flow Rate Source/LConn1 -- Thermal Mass/LConn1
  Convective Heat Transfer/RConn1 -- Heater Volume/LConn2
  Thermal Reference/LConn1 -- Controlled Heat Flow Rate Source/RConn2
  Heater Subsystem/RConn2 -- Controlled Heat Flow Rate Source/RConn1
  Flow Resistance (TL)/LConn1 -- Heater Volume/LConn1
  Flow Resistance (TL)1/RConn1 -- Heater Volume/RConn1
  Flow Resistance (TL)1/LConn1 -- A/RConn1
  Flow Resistance (TL)/RConn1 -- B/RConn1
  Controlled Current Source/LConn1 -- Electrical Reference/LConn1
  HV/RConn1 -- Voltage Sensor/LConn1 -- current sensing1/LConn1
  Controlled Current Source/RConn2 -- current sensing1/RConn1

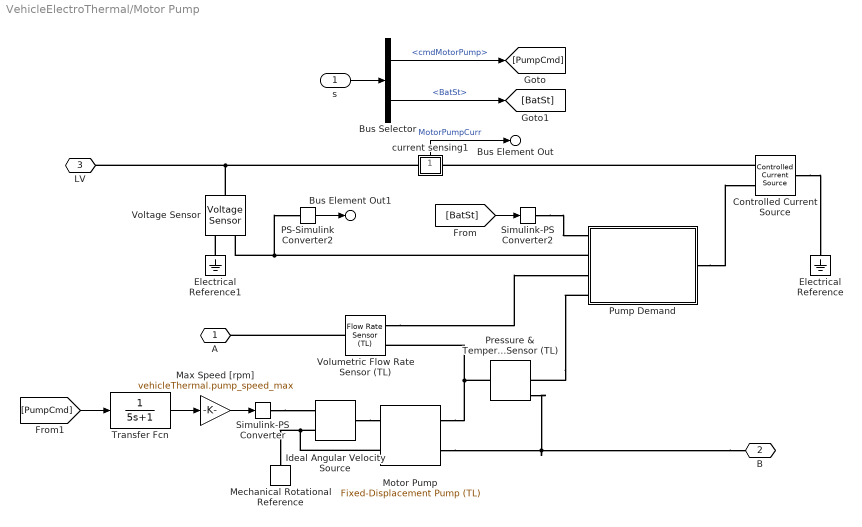
== system VehicleElectroThermal/Motor Pump ==
  s : Inport
  Bus Selector : BusSelector  OutputSignals=cmdMotorPump,BatSt
  Controlled Current Source : fl_lib/Electrical/Electrical Sources/Controlled Current Source
  Electrical Reference : fl_lib/Electrical/Electrical Elements/Electrical Reference
  Electrical Reference1 : fl_lib/Electrical/Electrical Elements/Electrical Reference
  Ideal Angular Velocity Source : fl_lib/Mechanical/Mechanical Sources/Ideal Angular Velocity Source
  Max Speed [rpm] : Gain  Gain=vehicleThermal.pump_speed_max
  Mechanical Rotational Reference : fl_lib/Mechanical/Rotational Elements/Mechanical Rotational Reference
  Motor Pump : SimscapeFluids_lib/Thermal Liquid/Pumps & Motors/Fixed-Displacement Pump (TL)  loss_spec=1  displacement=vehicleThermal.pump_displacement l/rev  omega_nominal=0.5 * vehicleThermal.pump_speed_max rpm  p_nominal=0.1 MPa  mu_nominal=0.9 cP  vol_eff_nominal=0.92  mech_eff_nominal=1/(1 + (0.6)/(vehicleThermal.pump_displacement)*0.006283185307179586 + (0.05)/(vehicleThermal.pump_displacement)/(0.1)*0.006283185307179586)  no_load_torque=0.05 N*m  p_diff_eff_TLU=[.1, 1, 2] MPa  omega_eff_TLU=[25, 50, 100, 200, 300, 400] rad/s  vol_eff_TLU=[.816, .908, .954, .977, .981, .984; .325, .663, .831, .916, .925, .946; .137, .568, .78, .892, .893, .91]  mech_eff_TLU=[.996, .996, .996, .996, .996, .996; .988, .989, .989, .989, .989, .99; .981, .981, .982, .982, .983, .984]  p_diff_loss_TLU=[.1, 1, 2] MPa  omega_loss_TLU=[25, 50, 100, 200, 300, 400] rad/s  vol_loss_TLU=[.023, .023, .023, .023, .0285, .032; .0844, .0842, .0845, .084, .1125, .108; .1079, .108, .11, .108, .1605, .18] * 1e-3 m^3/s  mech_loss_TLU=[.002, .002, .002, .002, .002, .002; .0607, .0556, .0556, .0556, .0556, .0505; .1937, .1937, .1833, .1833, .1729, .1626] N*m  vol_eff_min=1e-3  vol_eff_max=1  mech_eff_min=1e-3  mech_eff_max=1  pressure_threshold=1e-3 MPa  omega_threshold=10 rad/s  area=pi * vehicleThermal.coolant_pipe_D^2 / 4 m^2  quadrant_check=0  pump_mode_check=simscape.enum.assert.action.none
  PS-Simulink Converter2 : nesl_utility/PS-Simulink Converter  PhysicalDomain=network_engine_domain  SubClassName=ps_output  LeftPortType=input  RightPortType=output  PseudoPeriodic=off  Frequencies=[]  VectorFormat=inherit  Unit=inherit  AffineConversion=off
  Pressure & Temperature Sensor (TL) : fl_lib/Thermal Liquid/Sensors/Pressure & Temperature Sensor (TL)  reference=foundation.enum.MeasurementReference.difference  pressure=true  pressure_spec=foundation.enum.PressureMeasementSpec.Absolute  temperature=true
      settings: InternalSimscapePortConfiguration="{\"Bottom\":[{\"id\":\"T\",\"label\":\"T\",\"type\":\"output\"}],\"Left\":[{\"id\":\"A\",\"label\":\"A\",\"type\":\"foundation.thermal_liquid.thermal_liquid\"}],\"Right\":[{\"id\":\"B\",\"label\":\"B\",\"type\":\"foundation.thermal_liquid.thermal_liquid\"},{\"id\":\"P\",\"label\":\"P\",\"type\":\"output\"}],\"Top\":[]}"
  Pump Demand : Subsystem
  Simulink-PS Converter : nesl_utility/Simulink-PS Converter  PhysicalDomain=network_engine_domain  SubClassName=ps_input  LeftPortType=input  RightPortType=output  PseudoPeriodic=off  Frequencies=[]  NoiseDistribution=none  NoiseParameters=[]  Unit=rpm  AffineConversion=off  FilteringAndDerivatives=provide  SimscapeFilterOrder=1  InputFilterTimeConstant=0.001  UdotUserProvided=0
  Simulink-PS Converter2 : nesl_utility/Simulink-PS Converter  PhysicalDomain=network_engine_domain  SubClassName=ps_input  LeftPortType=input  RightPortType=output  PseudoPeriodic=off  Frequencies=[]  NoiseDistribution=none  NoiseParameters=[]  Unit=1  AffineConversion=off  FilteringAndDerivatives=provide  SimscapeFilterOrder=1  InputFilterTimeConstant=0.001  UdotUserProvided=0
  Transfer Fcn : TransferFcn  Denominator=[5 1]
  Voltage Sensor : fl_lib/Electrical/Electrical Sensors/Voltage Sensor
  Volumetric Flow Rate Sensor (TL) : fl_lib/Thermal Liquid/Sensors/Flow Rate Sensor (TL)  mass_flow_measure=false  volumetric_flow_measure=true  energy_flow_measure=false
      settings: InternalSimscapePortConfiguration="{\"Bottom\":[],\"Left\":[{\"id\":\"A\",\"label\":\"A\",\"type\":\"foundation.thermal_liquid.thermal_liquid\"}],\"Right\":[{\"id\":\"B\",\"label\":\"B\",\"type\":\"foundation.thermal_liquid.thermal_liquid\"},{\"id\":\"V\",\"label\":\"V\",\"type\":\"output\"}],\"Top\":[]}"
  current sensing1 : Subsystem
      settings: PortSchema="{\"entries\":[{\"content\":{\"sides\":[{\"content\":{\"connectorIds\":[\"LConn1\"]},\"type\":\"ConnectorPlacement.EquallySpacedRectSide\",\"uuid\":\"be2815b5-7c4b-4452-9f46-9765620d338b\"},{\"content\":{\"connectorIds\":[\"RConn1\"],\"side\":\"RIGHT\"},\"type\":\"ConnectorPlacement.EquallySpacedRectSide\",\"uuid\":\"398ebab2-f4fa-4d00-bf6e-74bf1f6972c5\"},{\"content\":{\"connectorIds\":[\"Out1\"],\"side\":\"TOP\"},\"type\":\"ConnectorPlacement.EquallySpacedRectSide\",\"uuid\":\"f18d5713-17ec-4be9-9072-3e03c5a4f599\"}]},\"type\":\"ConnectorPlacement.EquallySpacedConnector\",\"uuid\":\"966ec05e-6316-4039-8e26-1d6b096cf423\"}],\"packageUris\":[\"http://schema.mathworks.com/mf0/Connector/R2020b\"],\"version\":\"1.0\"}"
  A : PMIOPort  Side=Left
  B : PMIOPort  Port=2  Side=Right
  LV : PMIOPort  Port=3  Side=Right
  Bus Element Out : Outport  PortName=m  Element=MotorPumpCurr
  Bus Element Out1 : Outport  PortName=m  Element=LowVolt
  wires:
  [PumpCmd] -> Transfer Fcn/1
  [BatSt] -> Simulink-PS Converter2/1
  Bus Selector/2 -> [BatSt]  "<BatSt>"
  Bus Selector/1 -> [PumpCmd]  "<cmdMotorPump>"
  current sensing1/1("   ") -> Bus Element Out/1  "MotorPumpCurr"
  PS-Simulink Converter2/1 -> Bus Element Out1/1
  Transfer Fcn/1 -> Max Speed [rpm]/1
  Max Speed [rpm]/1 -> Simulink-PS Converter/1
  s/1 -> Bus Selector/1
  connections:
  Pump Demand/LConn4 -- Pressure & Temperature Sensor (TL)/RConn2
  Volumetric Flow Rate Sensor (TL)/RConn2 -- Pump Demand/LConn3
  Simulink-PS Converter2/RConn1 -- Pump Demand/LConn1
  Pump Demand/RConn1 -- Controlled Current Source/RConn1
  Volumetric Flow Rate Sensor (TL)/LConn1 -- A/RConn1
  Electrical Reference1/LConn1 -- Voltage Sensor/RConn2
  Voltage Sensor/RConn1 -- PS-Simulink Converter2/LConn1 -- Pump Demand/LConn2
  Controlled Current Source/LConn1 -- Electrical Reference/LConn1
  Controlled Current Source/RConn2 -- current sensing1/RConn1
  LV/RConn1 -- current sensing1/LConn1 -- Voltage Sensor/LConn1
  Ideal Angular Velocity Source/LConn1 -- Motor Pump/RConn1
  Motor Pump/RConn2 -- Mechanical Rotational Reference/LConn1 -- Ideal Angular Velocity Source/RConn2
  Simulink-PS Converter/RConn1 -- Ideal Angular Velocity Source/RConn1
  Volumetric Flow Rate Sensor (TL)/RConn1 -- Pressure & Temperature Sensor (TL)/LConn1 -- Motor Pump/LConn1
  B/RConn1 -- Pressure & Temperature Sensor (TL)/RConn1 -- Motor Pump/LConn2
